simulink model "sfcndemo_timestwo_for"  (Simulink 7.6)
settings: Solver=ode1  StartTime=0.0  StopTime=10.0  FixedStep=0.1  RelTol=1e-3
Description:
  | Simple Fortran S-function
settings Model: Creator=The MathWorks Inc.  CovMetricSettings=d  ExtModeAutoUpdateStatusClock=off
settings OptimizationCC: BlockReduction=off  BooleanDataType=off  InlineInvariantSignals=on  InitFltsAndDblsToZero=on
settings DebuggingCC: SaveWithParameterizedLinksMsg=none  SignalResolutionControl=TryResolveAllWithWarning  SolverPrmCheckMsg=none  MultiTaskDSMMsg=warning  MultiTaskCondExecSysMsg=none
settings HardwareCC: TargetUnknown=on
settings RTWCC: IncludeERTFirstTime=on
settings CodeAppCC: CustomSymbolStrFcn=$F$N$M
settings GRTTargetCC: TargetFcnLib=ansi_tfl_tmw.mat

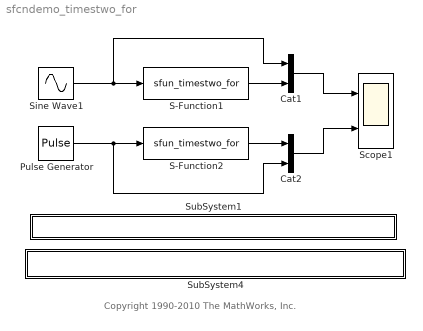
== system sfcndemo_timestwo_for ==
  note: Copyright 1990-2010 The MathWorks, Inc.
  Cat1 : Concatenate  Mode=Vector
  Cat2 : Concatenate  Mode=Vector
  Pulse Generator : DiscretePulseGenerator  PulseType=Time based  Amplitude=2  Period=1  PulseWidth=50
  S-Function1 : S-Function  FunctionName=sfun_timestwo_for  EnableBusSupport=off
  S-Function2 : S-Function  FunctionName=sfun_timestwo_for  EnableBusSupport=off
  Scope1 : Scope  NumInputPorts=2
      settings: TimeRange=10  YMin=-8~-1  YMax=8~5
  Sine Wave1 : Sin  Amplitude=3  SampleTime=0
  SubSystem1 : Subsystem  mask{filename=sfun_timestwo_for.F}
      mask init:
      | x=sfundemo_maskdisp;
      settings: AttributesFormatString=\n  OpenFcn=sfundemo_openfcn
      mask Display: disp(x);
  SubSystem4 : Subsystem  mask{filename=sfun_timestwo_for.tlc}
      mask init:
      | x=sfundemo_maskdisp;
      settings: AttributesFormatString=\n  OpenFcn=sfundemo_openfcn
      mask Display: disp(x);
  wires:
  Sine Wave1/1 -> S-Function1/1, Cat1/1
  S-Function1/1 -> Cat1/2
  S-Function2/1 -> Cat2/1
  Cat1/1 -> Scope1/1
  Cat2/1 -> Scope1/2
  Pulse Generator/1 -> S-Function2/1, Cat2/2

== system sfcndemo_timestwo_for/SubSystem1 ==

== system sfcndemo_timestwo_for/SubSystem4 ==
